simulink model "small_circuit_03"  (Simulink 10.0)
settings: Solver=ode45  StartTime=0.0  StopTime=20  RelTol=1e-3  EnableMultiTasking=on
settings Model: Creator=UX31  LastModifiedBy=unknown
settings DataIOCC: LimitDataPoints=on
settings DebuggingCC: UnderspecifiedInitializationDetection=Simplified  MergeDetectMultiDrivingBlocksExec=error  SolverPrmCheckMsg=warning
settings GRTTargetCC: GeneratePreprocessorConditionals=Disable all  CombineOutputUpdateFcns=on  GRTInterface=off
settings ConfigComp: CovExternalEMLEnable=off  CovSFcnEnable=off

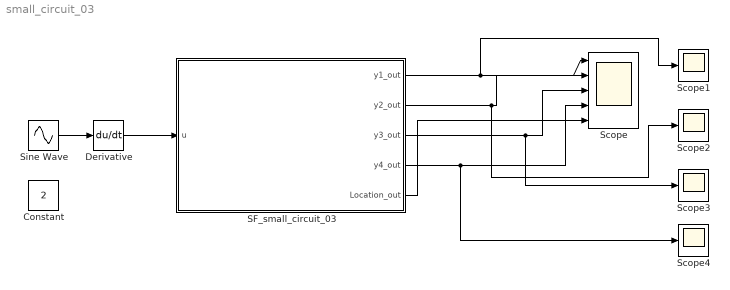
== system small_circuit_03 ==
  Constant : Constant  Value=2
  Derivative : Derivative
  SF_small_circuit_03 : Stateflow chart  TreatAsAtomicUnit=on
  Scope : Scope  NumInputPorts=5
  Scope{1..4} (4 alike) : Scope
  Sine Wave : Sin  SampleTime=0
  wires:
  SF_small_circuit_03/1(y1_out) -> Scope1/1, Scope/1
  SF_small_circuit_03/2(y2_out) -> Scope2/1, Scope/2
  SF_small_circuit_03/3(y3_out) -> Scope3/1, Scope/3
  SF_small_circuit_03/4(y4_out) -> Scope4/1, Scope/4
  SF_small_circuit_03/5(Location_out) -> Scope/5
  Derivative/1 -> SF_small_circuit_03/1(u)
  Sine Wave/1 -> Derivative/1

== stateflow chart SF_small_circuit_03 ==
  settings: updateMethod=CONTINUOUS
  state always
    du:
    y1_dot=0-y3;
    y2_dot=y1;
    y3_dot=y1-y3-u;
    y4_dot=0-y3;
    y1_out=y1;
    y2_out=y2;
    y3_out=y3;
    y4_out=y4;
    Location_out =1;
  (default) -> always : {y1=0;y2=0;y3=0;y4=0}
  data: y1 local double; y1_out output double; y2 local double; y2_out output double; y3 local double; y3_out output double; y4 local double; y4_out output double; Location_out output double; u input double
  data y1 settings: updateMethod=SF_CONTINUOUS_TIME_DATA
  data y2 settings: updateMethod=SF_CONTINUOUS_TIME_DATA
  data y3 settings: updateMethod=SF_CONTINUOUS_TIME_DATA
  data y4 settings: updateMethod=SF_CONTINUOUS_TIME_DATA
